simulink model "FPU_integrator_gen"  (Simulink 7.6)
settings: Solver=FixedStepDiscrete  StartTime=0.0  StopTime=50  FixedStep=1  RelTol=1e-3
libraries: simulink x6
settings Model: Creator=jordan  LastModifiedBy=jordan
settings OptimizationCC: BlockReduction=off  ConditionallyExecuteInputs=off

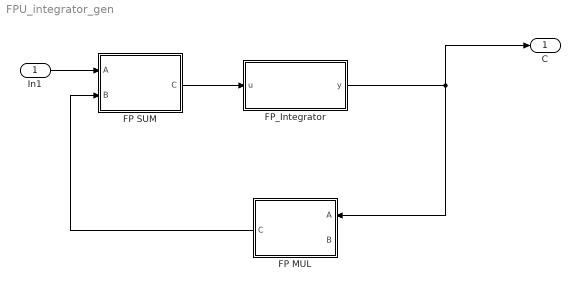
== system FPU_integrator_gen ==
  In1 : Inport
  FP MUL : Subsystem
  FP SUM : Subsystem
  FP_Integrator : Subsystem
  C : Outport  InitialOutput=0
  wires:
  FP_Integrator/1(y) -> C/1, FP MUL/1(A)
  In1/1 -> FP SUM/1(A)
  FP SUM/1(C) -> FP_Integrator/1(u)
  FP MUL/1(C) -> FP SUM/2(B)

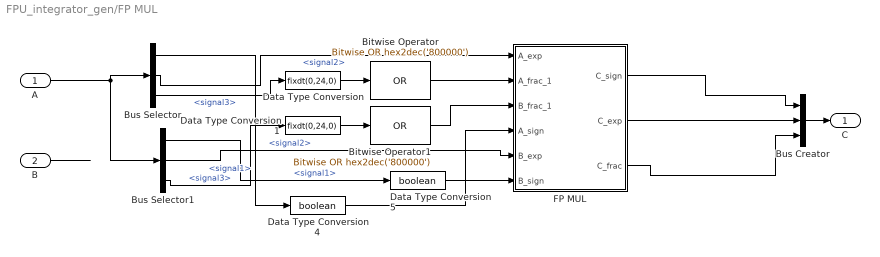
== system FPU_integrator_gen/FP MUL ==
  A : Inport
  B : Inport  Port=2
  Bitwise Operator : simulink/Logic and Bit Operations/Bitwise Operator  logicop=OR  UseBitMask=on  BitMask=hex2dec('800000')  BitMaskRealWorld=Stored Integer
  Bitwise Operator1 : simulink/Logic and Bit Operations/Bitwise Operator  logicop=OR  UseBitMask=on  BitMask=hex2dec('800000')  BitMaskRealWorld=Stored Integer
  Bus Creator : BusCreator  Inputs=3
  Bus Selector : BusSelector  OutputSignals=signal1,signal2,signal3
  Bus Selector1 : BusSelector  OutputSignals=signal1,signal2,signal3
  Data Type Conversion : DataTypeConversion  OutDataTypeStr=fixdt(0,24,0)  RndMeth=Nearest
  Data Type Conversion1 : DataTypeConversion  OutDataTypeStr=fixdt(0,24,0)  RndMeth=Nearest
  Data Type Conversion4 : DataTypeConversion  OutDataTypeStr=boolean  RndMeth=Nearest
  Data Type Conversion5 : DataTypeConversion  OutDataTypeStr=boolean  RndMeth=Nearest
  FP MUL : Subsystem
  C : Outport  InitialOutput=0
  wires:
  Data Type Conversion5/1 -> FP MUL/6(B_sign)
  Data Type Conversion4/1 -> FP MUL/4(A_sign)
  FP MUL/3(C_frac) -> Bus Creator/3
  FP MUL/2(C_exp) -> Bus Creator/2
  FP MUL/1(C_sign) -> Bus Creator/1
  Bitwise Operator1/1 -> FP MUL/3(B_frac_1)
  Data Type Conversion1/1 -> Bitwise Operator1/1
  Bitwise Operator/1 -> FP MUL/2(A_frac_1)
  Data Type Conversion/1 -> Bitwise Operator/1
  Bus Selector1/3 -> Data Type Conversion1/1  "<signal3>"
  Bus Selector/3 -> Data Type Conversion/1  "<signal3>"
  Bus Selector1/2 -> FP MUL/5(B_exp)  "<signal2>"
  Bus Selector/2 -> FP MUL/1(A_exp)  "<signal2>"
  Bus Selector1/1 -> Data Type Conversion5/1  "<signal1>"
  Bus Selector/1 -> Data Type Conversion4/1  "<signal1>"
  B/1 -> ?
  A/1 -> Bus Selector/1, Bus Selector1/1
  Bus Creator/1 -> C/1

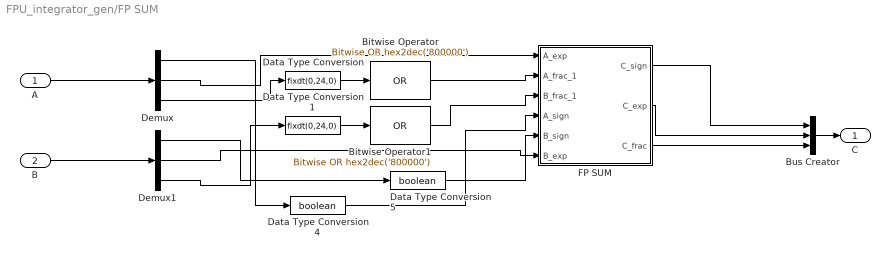
== system FPU_integrator_gen/FP SUM ==
  A : Inport
  B : Inport  Port=2
  Bitwise Operator : simulink/Logic and Bit Operations/Bitwise Operator  logicop=OR  UseBitMask=on  BitMask=hex2dec('800000')  BitMaskRealWorld=Stored Integer
  Bitwise Operator1 : simulink/Logic and Bit Operations/Bitwise Operator  logicop=OR  UseBitMask=on  BitMask=hex2dec('800000')  BitMaskRealWorld=Stored Integer
  Bus Creator : BusCreator  Inputs=3
  Data Type Conversion : DataTypeConversion  OutDataTypeStr=fixdt(0,24,0)  RndMeth=Nearest
  Data Type Conversion1 : DataTypeConversion  OutDataTypeStr=fixdt(0,24,0)  RndMeth=Nearest
  Data Type Conversion4 : DataTypeConversion  OutDataTypeStr=boolean  RndMeth=Nearest
  Data Type Conversion5 : DataTypeConversion  OutDataTypeStr=boolean  RndMeth=Nearest
  Demux : Demux  Outputs=3
  Demux1 : Demux  Outputs=3
  FP SUM : Subsystem
  C : Outport  PortDimensions=3  InitialOutput=0
  wires:
  A/1 -> Demux/1
  B/1 -> Demux1/1
  Demux/1 -> Data Type Conversion4/1
  Demux1/1 -> Data Type Conversion5/1
  Demux/2 -> FP SUM/1(A_exp)
  Demux1/2 -> FP SUM/6(B_exp)
  Demux/3 -> Data Type Conversion/1
  Demux1/3 -> Data Type Conversion1/1
  Data Type Conversion/1 -> Bitwise Operator/1
  Bitwise Operator/1 -> FP SUM/2(A_frac_1)
  Data Type Conversion1/1 -> Bitwise Operator1/1
  Bitwise Operator1/1 -> FP SUM/3(B_frac_1)
  FP SUM/1(C_sign) -> Bus Creator/1
  FP SUM/2(C_exp) -> Bus Creator/2
  FP SUM/3(C_frac) -> Bus Creator/3
  Data Type Conversion4/1 -> FP SUM/4(A_sign)
  Data Type Conversion5/1 -> FP SUM/5(B_sign)
  Bus Creator/1 -> C/1

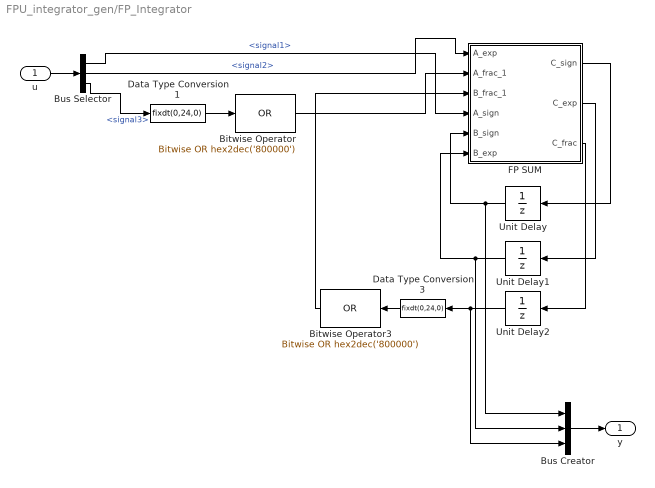
== system FPU_integrator_gen/FP_Integrator ==
  u : Inport
  Bitwise Operator : simulink/Logic and Bit Operations/Bitwise Operator  logicop=OR  UseBitMask=on  BitMask=hex2dec('800000')  BitMaskRealWorld=Stored Integer
  Bitwise Operator3 : simulink/Logic and Bit Operations/Bitwise Operator  logicop=OR  UseBitMask=on  BitMask=hex2dec('800000')  BitMaskRealWorld=Stored Integer
  Bus Creator : BusCreator  Inputs=3
  Bus Selector : BusSelector  OutputSignals=signal1,signal2,signal3
  Data Type Conversion1 : DataTypeConversion  OutDataTypeStr=fixdt(0,24,0)  RndMeth=Nearest
  Data Type Conversion3 : DataTypeConversion  OutDataTypeStr=fixdt(0,24,0)  RndMeth=Nearest
  FP SUM : Subsystem
  Unit Delay : UnitDelay  SampleTime=-1
  Unit Delay1 : UnitDelay  SampleTime=-1
  Unit Delay2 : UnitDelay  SampleTime=-1
  y : Outport
  wires:
  FP SUM/1(C_sign) -> Unit Delay/1
  FP SUM/2(C_exp) -> Unit Delay1/1
  FP SUM/3(C_frac) -> Unit Delay2/1
  Unit Delay/1 -> FP SUM/5(B_sign), Bus Creator/1
  Unit Delay1/1 -> FP SUM/6(B_exp), Bus Creator/2
  Unit Delay2/1 -> Data Type Conversion3/1, Bus Creator/3
  Data Type Conversion3/1 -> Bitwise Operator3/1
  Bitwise Operator3/1 -> FP SUM/3(B_frac_1)
  Bus Selector/1 -> FP SUM/4(A_sign)  "<signal1>"
  Bus Selector/2 -> FP SUM/1(A_exp)  "<signal2>"
  Data Type Conversion1/1 -> Bitwise Operator/1
  Bus Selector/3 -> Data Type Conversion1/1  "<signal3>"
  Bitwise Operator/1 -> FP SUM/2(A_frac_1)
  u/1 -> Bus Selector/1
  Bus Creator/1 -> y/1

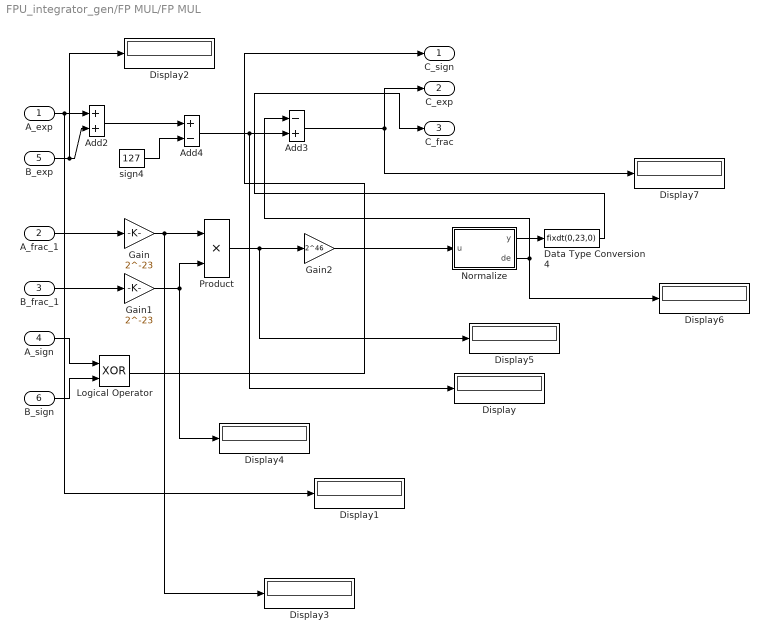
== system FPU_integrator_gen/FP MUL/FP MUL ==
  A_exp : Inport  OutDataTypeStr=uint8
  A_frac_1 : Inport  Port=2  OutDataTypeStr=fixdt(0,24,0)
  B_frac_1 : Inport  Port=3  OutDataTypeStr=fixdt(0,24,0)
  A_sign : Inport  Port=4  OutDataTypeStr=boolean
  B_exp : Inport  Port=5  OutDataTypeStr=uint8
  B_sign : Inport  Port=6  OutDataTypeStr=boolean
  Add2 : Sum  OutDataTypeStr=fixdt(0,9,0)  RndMeth=Nearest
  Add3 : Sum  Inputs=-+  OutDataTypeStr=uint8  RndMeth=Nearest  SaturateOnIntegerOverflow=on
  Add4 : Sum  Inputs=+-  OutDataTypeStr=uint8  RndMeth=Nearest  SaturateOnIntegerOverflow=on
  Data Type Conversion4 : DataTypeConversion  OutDataTypeStr=fixdt(0,23,0)
  Display{,1..7} (8 alike) : Display
  Gain : Gain  Gain=2^-23  OutDataTypeStr=fixdt(0,24,23)  RndMeth=Nearest
  Gain1 : Gain  Gain=2^-23  OutDataTypeStr=fixdt(0,24,23)  RndMeth=Nearest
  Gain2 : Gain  Gain=2^46  OutDataTypeStr=fixdt(0,48,0)  RndMeth=Nearest
  Logical Operator : Logic  Operator=XOR  AllPortsSameDT=off  OutDataTypeStr=boolean
  Normalize : Stateflow chart  TreatAsAtomicUnit=on
  Product : Product  OutDataTypeStr=fixdt(0,48,46)  RndMeth=Nearest
  sign4 : Constant  Value=127  OutDataTypeStr=fixdt(0,9,0)
  C_sign : Outport  OutDataTypeStr=boolean
  C_exp : Outport  Port=2  OutDataTypeStr=uint8
  C_frac : Outport  Port=3  OutDataTypeStr=fixdt(0,23,0)
  wires:
  Gain2/1 -> Normalize/1(u)
  B_sign/1 -> Logical Operator/2
  A_exp/1 -> Display1/1, Add2/1
  A_sign/1 -> Logical Operator/1
  B_frac_1/1 -> Gain1/1
  A_frac_1/1 -> Gain/1
  Gain1/1 -> Display4/1, Product/2
  Gain/1 -> Display3/1, Product/1
  Add4/1 -> Display/1, Add3/2
  sign4/1 -> Add4/2
  Add2/1 -> Add4/1
  Product/1 -> Gain2/1, Display5/1
  Logical Operator/1 -> C_sign/1
  Data Type Conversion4/1 -> C_frac/1
  Add3/1 -> Display7/1, C_exp/1
  Normalize/2(de) -> Display6/1, Add3/1
  Normalize/1(y) -> Data Type Conversion4/1
  B_exp/1 -> Display2/1, Add2/2

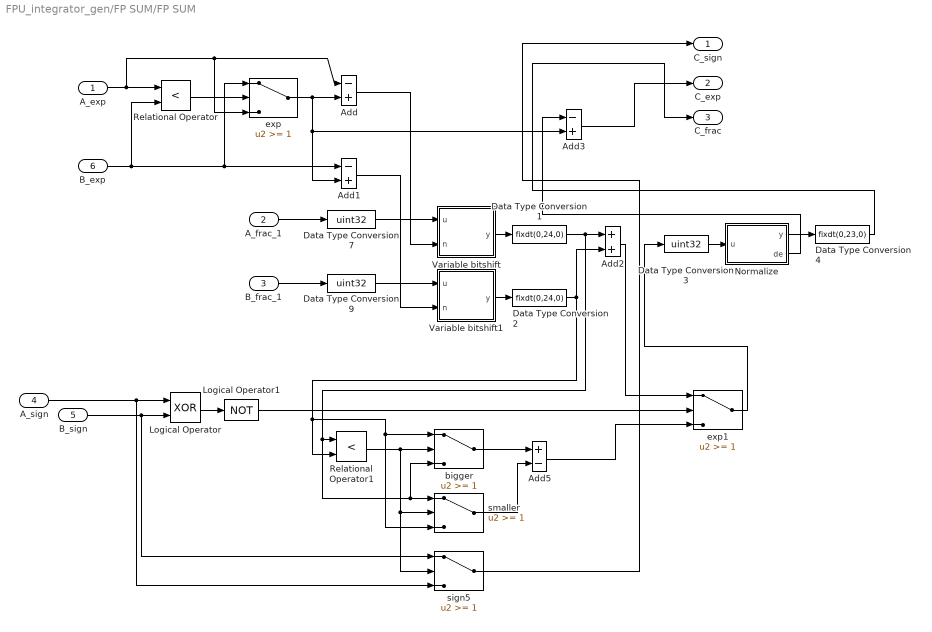
== system FPU_integrator_gen/FP SUM/FP SUM ==
  A_exp : Inport  OutDataTypeStr=uint8
  A_frac_1 : Inport  Port=2  OutDataTypeStr=fixdt(0,24,0)
  B_frac_1 : Inport  Port=3  OutDataTypeStr=fixdt(0,24,0)
  A_sign : Inport  Port=4  OutDataTypeStr=boolean
  B_sign : Inport  Port=5  OutDataTypeStr=boolean
  B_exp : Inport  Port=6  OutDataTypeStr=uint8
  Add : Sum  Inputs=-+  OutDataTypeStr=int8
  Add1 : Sum  Inputs=-+  OutDataTypeStr=int8
  Add2 : Sum  OutDataTypeStr=fixdt(0,25,0)  RndMeth=Nearest
  Add3 : Sum  Inputs=-+  OutDataTypeStr=uint8  SaturateOnIntegerOverflow=on
  Add5 : Sum  Inputs=+-  OutDataTypeStr=fixdt(0,25,0)  RndMeth=Nearest
  Data Type Conversion1 : DataTypeConversion  OutDataTypeStr=fixdt(0,24,0)
  Data Type Conversion2 : DataTypeConversion  OutDataTypeStr=fixdt(0,24,0)
  Data Type Conversion3 : DataTypeConversion  OutDataTypeStr=uint32
  Data Type Conversion4 : DataTypeConversion  OutDataTypeStr=fixdt(0,23,0)
  Data Type Conversion7 : DataTypeConversion  OutDataTypeStr=uint32
  Data Type Conversion9 : DataTypeConversion  OutDataTypeStr=uint32
  Logical Operator : Logic  Operator=XOR  AllPortsSameDT=off  OutDataTypeStr=boolean
  Logical Operator1 : Logic  Operator=NOT  AllPortsSameDT=off  OutDataTypeStr=boolean
  Normalize : Stateflow chart  TreatAsAtomicUnit=on
  Relational Operator : RelationalOperator  Operator=<  OutDataTypeStr=boolean
  Relational Operator1 : RelationalOperator  Operator=<  OutDataTypeStr=boolean
  Variable bitshift : Stateflow chart  TreatAsAtomicUnit=on
  Variable bitshift1 : Stateflow chart  TreatAsAtomicUnit=on
  bigger : Switch  Threshold=1
  exp : Switch  Threshold=1
  exp1 : Switch  Threshold=1
  sign5 : Switch  Threshold=1
  smaller : Switch  Threshold=1
  C_sign : Outport  OutDataTypeStr=boolean
  C_exp : Outport  Port=2  OutDataTypeStr=uint8
  C_frac : Outport  Port=3  OutDataTypeStr=fixdt(0,23,0)
  wires:
  Add3/1 -> C_exp/1
  B_sign/1 -> sign5/1, Logical Operator/2
  A_sign/1 -> sign5/3, Logical Operator/1
  Data Type Conversion9/1 -> Variable bitshift1/1(u)
  Data Type Conversion7/1 -> Variable bitshift/1(u)
  sign5/1 -> C_sign/1
  exp1/1 -> Data Type Conversion3/1
  Add5/1 -> exp1/3
  smaller/1 -> Add5/2
  bigger/1 -> Add5/1
  Relational Operator1/1 -> sign5/2, smaller/2, bigger/2
  Logical Operator1/1 -> exp1/2
  Logical Operator/1 -> Logical Operator1/1
  Data Type Conversion4/1 -> C_frac/1
  Data Type Conversion3/1 -> Normalize/1(u)
  Normalize/2(de) -> Add3/1
  Normalize/1(y) -> Data Type Conversion4/1
  Add2/1 -> exp1/1
  Data Type Conversion2/1 -> smaller/3, bigger/1, Relational Operator1/2, Add2/2
  Variable bitshift1/1(y) -> Data Type Conversion2/1
  Add1/1 -> Variable bitshift1/2(n)
  Add/1 -> Variable bitshift/2(n)
  B_frac_1/1 -> Data Type Conversion9/1
  exp/1 -> Add3/2, Add1/2, Add/2
  Relational Operator/1 -> exp/2
  Data Type Conversion1/1 -> bigger/3, smaller/1, Relational Operator1/1, Add2/1
  Variable bitshift/1(y) -> Data Type Conversion1/1
  A_frac_1/1 -> Data Type Conversion7/1
  B_exp/1 -> Relational Operator/2, Add1/1, exp/1
  A_exp/1 -> Add/1, exp/3, Relational Operator/1

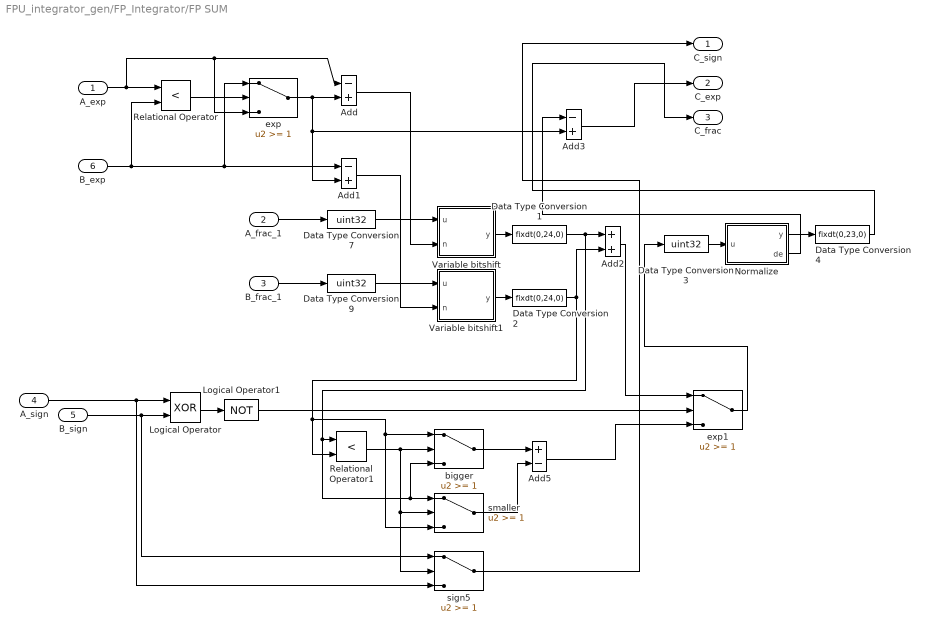
== system FPU_integrator_gen/FP_Integrator/FP SUM ==
  A_exp : Inport  OutDataTypeStr=uint8
  A_frac_1 : Inport  Port=2  OutDataTypeStr=fixdt(0,24,0)
  B_frac_1 : Inport  Port=3  OutDataTypeStr=fixdt(0,24,0)
  A_sign : Inport  Port=4  OutDataTypeStr=boolean
  B_sign : Inport  Port=5  OutDataTypeStr=boolean
  B_exp : Inport  Port=6  OutDataTypeStr=uint8
  Add : Sum  Inputs=-+  OutDataTypeStr=int8
  Add1 : Sum  Inputs=-+  OutDataTypeStr=int8
  Add2 : Sum  OutDataTypeStr=fixdt(0,25,0)  RndMeth=Nearest
  Add3 : Sum  Inputs=-+  OutDataTypeStr=uint8  SaturateOnIntegerOverflow=on
  Add5 : Sum  Inputs=+-  OutDataTypeStr=fixdt(0,25,0)  RndMeth=Nearest
  Data Type Conversion1 : DataTypeConversion  OutDataTypeStr=fixdt(0,24,0)
  Data Type Conversion2 : DataTypeConversion  OutDataTypeStr=fixdt(0,24,0)
  Data Type Conversion3 : DataTypeConversion  OutDataTypeStr=uint32
  Data Type Conversion4 : DataTypeConversion  OutDataTypeStr=fixdt(0,23,0)
  Data Type Conversion7 : DataTypeConversion  OutDataTypeStr=uint32
  Data Type Conversion9 : DataTypeConversion  OutDataTypeStr=uint32
  Logical Operator : Logic  Operator=XOR  AllPortsSameDT=off  OutDataTypeStr=boolean
  Logical Operator1 : Logic  Operator=NOT  AllPortsSameDT=off  OutDataTypeStr=boolean
  Normalize : Stateflow chart  TreatAsAtomicUnit=on
  Relational Operator : RelationalOperator  Operator=<  OutDataTypeStr=boolean
  Relational Operator1 : RelationalOperator  Operator=<  OutDataTypeStr=boolean
  Variable bitshift : Stateflow chart  TreatAsAtomicUnit=on
  Variable bitshift1 : Stateflow chart  TreatAsAtomicUnit=on
  bigger : Switch  Threshold=1
  exp : Switch  Threshold=1
  exp1 : Switch  Threshold=1
  sign5 : Switch  Threshold=1
  smaller : Switch  Threshold=1
  C_sign : Outport  OutDataTypeStr=boolean
  C_exp : Outport  Port=2  OutDataTypeStr=uint8
  C_frac : Outport  Port=3  OutDataTypeStr=fixdt(0,23,0)
  wires:
  Add3/1 -> C_exp/1
  B_sign/1 -> sign5/1, Logical Operator/2
  A_sign/1 -> sign5/3, Logical Operator/1
  Data Type Conversion9/1 -> Variable bitshift1/1(u)
  Data Type Conversion7/1 -> Variable bitshift/1(u)
  sign5/1 -> C_sign/1
  exp1/1 -> Data Type Conversion3/1
  Add5/1 -> exp1/3
  smaller/1 -> Add5/2
  bigger/1 -> Add5/1
  Relational Operator1/1 -> sign5/2, smaller/2, bigger/2
  Logical Operator1/1 -> exp1/2
  Logical Operator/1 -> Logical Operator1/1
  Data Type Conversion4/1 -> C_frac/1
  Data Type Conversion3/1 -> Normalize/1(u)
  Normalize/2(de) -> Add3/1
  Normalize/1(y) -> Data Type Conversion4/1
  Add2/1 -> exp1/1
  Data Type Conversion2/1 -> smaller/3, bigger/1, Relational Operator1/2, Add2/2
  Variable bitshift1/1(y) -> Data Type Conversion2/1
  Add1/1 -> Variable bitshift1/2(n)
  Add/1 -> Variable bitshift/2(n)
  B_frac_1/1 -> Data Type Conversion9/1
  exp/1 -> Add3/2, Add1/2, Add/2
  Relational Operator/1 -> exp/2
  Data Type Conversion1/1 -> bigger/3, smaller/1, Relational Operator1/1, Add2/1
  Variable bitshift/1(y) -> Data Type Conversion1/1
  A_frac_1/1 -> Data Type Conversion7/1
  B_exp/1 -> Relational Operator/2, Add1/1, exp/1
  A_exp/1 -> Add/1, exp/3, Relational Operator/1

== matlab function FP_Integrator/FP SUM/Normalize ==
  data: u input uint32; y output uint32; de output double
function [y,de] = fcn(u)
%#eml

buf=u;
p=int8(-1);
c=bitand(buf,2^24);
for ind=1:25
    if (~c)
        p=p+1;
        buf=bitshift(buf,1);
        c=bitand(buf,2^24);
    end
end
bufy = bitand(bitshift(u,p),2^23-1);
y=bufy;
de=p;

== matlab function FP_Integrator/FP SUM/Variable bitshift ==
  data: u input uint32; y output uint32; n input int8
function y = fcn(u,n)
%#eml

y = bitshift(u,-n);

== matlab function FP_Integrator/FP SUM/Variable bitshift1 ==
  data: u input uint32; y output uint32; n input int8
function y = fcn(u,n)
%#eml

y = bitshift(u,-n);

== matlab function FP SUM/FP SUM/Normalize ==
  data: u input uint32; y output uint32; de output double
function [y,de] = fcn(u)
%#eml

buf=u;
p=int8(-1);
c=bitand(buf,2^24);
for ind=1:25
    if (~c)
        p=p+1;
        buf=bitshift(buf,1);
        c=bitand(buf,2^24);
    end
end
bufy = bitand(bitshift(u,p),2^23-1);
y=bufy;
de=p;

== matlab function FP MUL/FP MUL/Normalize ==
  data: u input fixdt(0,48,0); y output uint32; de output double
function [y,de] = fcn(u)
%#eml

buf=u;
p=int8(-1);
c=bitand(buf,fi(2^47,0,48,0));
for ind=1:25
    if (c==0)
        p=p+1;
        buf=bitshift(buf,1);
        c=bitand(buf,fi(2^47,0,48,0));
    end
end
bufy = bitand(bitshift(u,p),fi(2^46-1,0,48,0));
y=uint32(bitshift(bufy,-23));
de=p;

== matlab function FP SUM/FP SUM/Variable bitshift ==
  data: u input uint32; y output uint32; n input int8
function y = fcn(u,n)
%#eml

y = bitshift(u,-n);

== matlab function FP SUM/FP SUM/Variable bitshift1 ==
  data: u input uint32; y output uint32; n input int8
function y = fcn(u,n)
%#eml

y = bitshift(u,-n);
